simulink model "ebox2010"  (Simulink 7.5)
settings: Solver=FixedStepDiscrete  StartTime=0.0  StopTime=1000  FixedStep=1/1000  RelTol=1e-3
settings Model: Creator=root  LastModifiedBy=root  SimulationMode=external  ExtModeAutoUpdateStatusClock=off
settings OptimizationCC: InitFltsAndDblsToZero=on
settings DebuggingCC: SaveWithParameterizedLinksMsg=none  SignalResolutionControl=TryResolveAllWithWarning  MultiTaskDSMMsg=warning  MultiTaskCondExecSysMsg=none  StrictBusMsg=None
settings RTWCC: SystemTargetFile=ectarget.tlc  MakeCommand=make_rtw OPTS='-DNETIF_ID=0'  TemplateMakefile=ec_unix.tmf  Description=Ethercattarget Real-Time Target for PREEMPT-RT/Linux  ProcessScript=ectarget_make_rtw_hook  IncludeERTFirstTime=on
settings GRTTargetCC: TargetFcnLib=ansi_tfl_tmw.mat  ExtMode=on  ExtModeMexArgs='localhost'

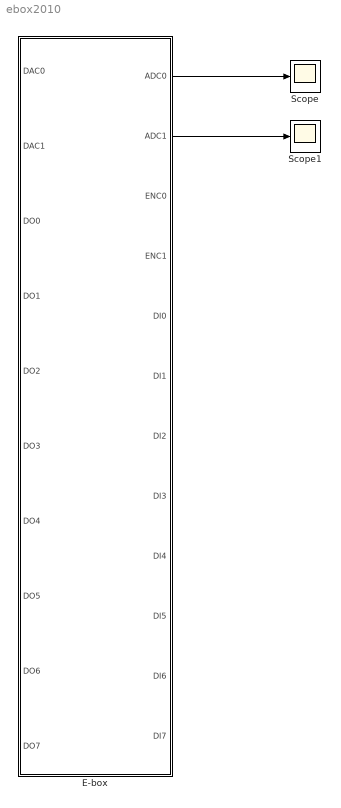
== system ebox2010 ==
  E-box : Subsystem  mask(E-box){link_id=0}
      mask prompts: link_id "Link id (>0)"
  Scope : Scope
      settings: TimeRange=0.2  YMin=0.0025  YMax=0.00675  SaveName=y1  DataFormat=Array
  Scope1 : Scope
      settings: TimeRange=1  YMin=-9  YMax=9  SaveName=y2  DataFormat=Array
  wires:
  E-box/1(ADC0) -> Scope/1
  E-box/2(ADC1) -> Scope1/1

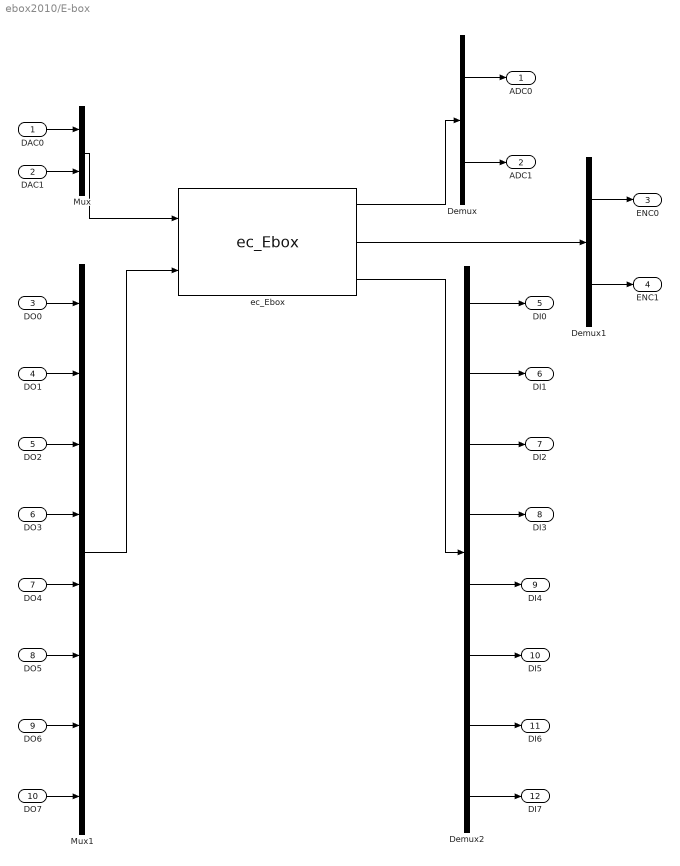
== system ebox2010/E-box ==
  DAC0 : Inport  OutDataType=sfix(16)  OutScaling=2^0
  DAC1 : Inport  Port=2  OutDataType=sfix(16)  OutScaling=2^0
  DO0 : Inport  Port=3  OutDataType=sfix(16)  OutScaling=2^0
  DO1 : Inport  Port=4  OutDataType=sfix(16)  OutScaling=2^0
  DO2 : Inport  Port=5  OutDataType=sfix(16)  OutScaling=2^0
  DO3 : Inport  Port=6  OutDataType=sfix(16)  OutScaling=2^0
  DO4 : Inport  Port=7  OutDataType=sfix(16)  OutScaling=2^0
  DO5 : Inport  Port=8  OutDataType=sfix(16)  OutScaling=2^0
  DO6 : Inport  Port=9  OutDataType=sfix(16)  OutScaling=2^0
  DO7 : Inport  Port=10  OutDataType=sfix(16)  OutScaling=2^0
  Demux : Demux  Outputs=2
  Demux1 : Demux  Outputs=2
  Demux2 : Demux  Outputs=8
  Mux : Mux  Inputs=2
  Mux1 : Mux  Inputs=8
  ec_Ebox : S-Function  FunctionName=ec_Ebox  Parameters=link_id  EnableBusSupport=off  mask{link_id=link_id}
      mask prompts: link_id "analog in id (start from 1)"
      mask Display:
      | port_label('output',1,'ADC')
      | port_label('output',2,'ENC')
      | port_label('output',3,'DI')
      | port_label('input',1,'DAC')
      | port_label('input',2,'DO')
  ADC0 : Outport  OutDataType=sfix(16)  OutScaling=2^0
  ADC1 : Outport  Port=2  OutDataType=sfix(16)  OutScaling=2^0
  ENC0 : Outport  Port=3  OutDataType=sfix(16)  OutScaling=2^0
  ENC1 : Outport  Port=4  OutDataType=sfix(16)  OutScaling=2^0
  DI0 : Outport  Port=5  OutDataType=sfix(16)  OutScaling=2^0
  DI1 : Outport  Port=6  OutDataType=sfix(16)  OutScaling=2^0
  DI2 : Outport  Port=7  OutDataType=sfix(16)  OutScaling=2^0
  DI3 : Outport  Port=8  OutDataType=sfix(16)  OutScaling=2^0
  DI4 : Outport  Port=9  OutDataType=sfix(16)  OutScaling=2^0
  DI5 : Outport  Port=10  OutDataType=sfix(16)  OutScaling=2^0
  DI6 : Outport  Port=11  OutDataType=sfix(16)  OutScaling=2^0
  DI7 : Outport  Port=12  OutDataType=sfix(16)  OutScaling=2^0
  wires:
  ec_Ebox/1 -> Demux/1
  Demux/1 -> ADC0/1
  Demux/2 -> ADC1/1
  Demux1/1 -> ENC0/1
  Demux1/2 -> ENC1/1
  ec_Ebox/2 -> Demux1/1
  Mux/1 -> ec_Ebox/1
  DAC0/1 -> Mux/1
  DAC1/1 -> Mux/2
  ec_Ebox/3 -> Demux2/1
  Demux2/1 -> DI0/1
  Demux2/2 -> DI1/1
  Demux2/3 -> DI2/1
  Demux2/4 -> DI3/1
  Demux2/5 -> DI4/1
  Demux2/6 -> DI5/1
  Demux2/7 -> DI6/1
  Demux2/8 -> DI7/1
  Mux1/1 -> ec_Ebox/2
  DO0/1 -> Mux1/1
  DO1/1 -> Mux1/2
  DO2/1 -> Mux1/3
  DO3/1 -> Mux1/4
  DO4/1 -> Mux1/5
  DO5/1 -> Mux1/6
  DO6/1 -> Mux1/7
  DO7/1 -> Mux1/8
